simulink model "lab2zad1"  (R2022b)
settings: Solver=VariableStepAuto  StartTime=0.0  StopTime=10  RelTol=1e-3
settings Model: Creator=User  LastModifiedBy=User

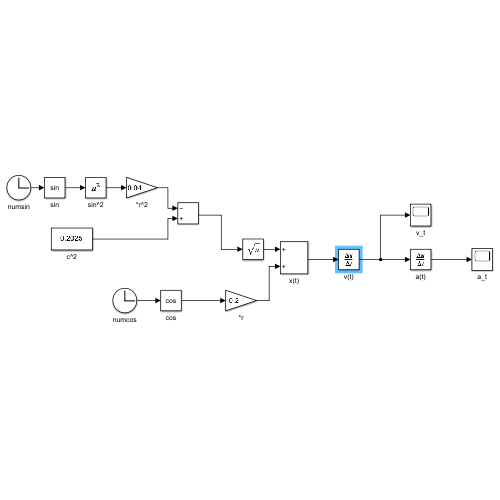
[thumbnail: Simulink's stored preview of the top-level diagram]
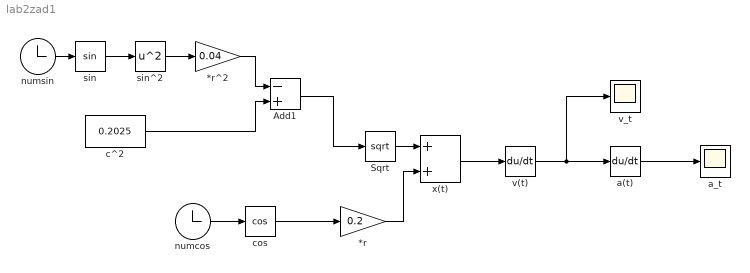
== system lab2zad1 ==
  *r : Gain  Gain=0.2
  *r^2 : Gain  Gain=0.04
  Add1 : Sum  Inputs=-+
  Sqrt : Sqrt
  a(t) : Derivative
  a_t : Scope
  c^2 : Constant  Value=0.2025
  cos : Trigonometry  Operator=cos
  numcos : Clock
  numsin : Clock
  sin : Trigonometry
  sin^2 : Math  Operator=square
  v(t) : Derivative
  v_t : Scope
  x(t) : Sum
  wires:
  numcos/1 -> cos/1
  cos/1 -> *r/1
  *r/1 -> x(t)/2
  c^2/1 -> Add1/2
  Sqrt/1 -> x(t)/1
  Add1/1 -> Sqrt/1
  numsin/1 -> sin/1
  sin/1 -> sin^2/1
  sin^2/1 -> *r^2/1
  *r^2/1 -> Add1/1
  x(t)/1 -> v(t)/1
  v(t)/1 -> a(t)/1, v_t/1
  a(t)/1 -> a_t/1
